simulink model "punto_cd_simulink_200901"  (R2019a)
settings: Solver=VariableStepAuto  StartTime=0.0  StopTime=36*2*pi  RelTol=1e-3
libraries: cstblocks x2
settings Model: Creator=Marco Greco  LastModifiedBy=Marco Greco

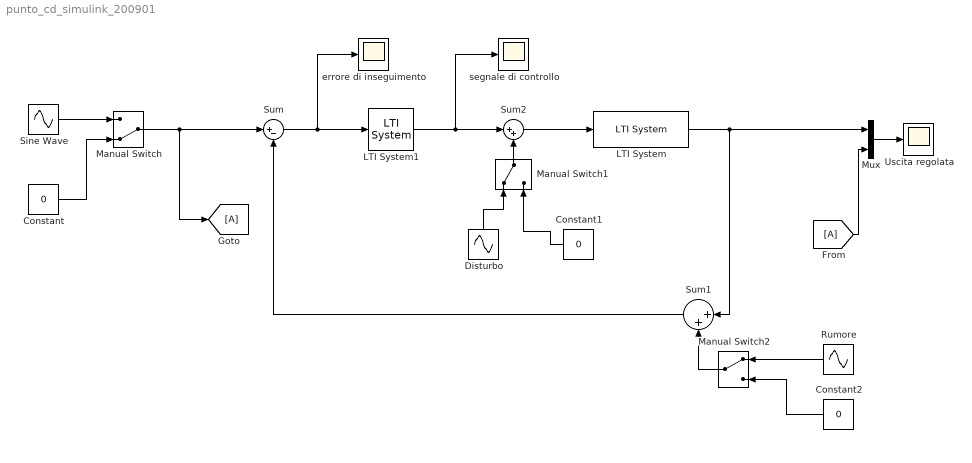
== system punto_cd_simulink_200901 ==
  " Disturbo" : Sin  Frequency=0.2  SampleTime=0
  Constant : Constant  Value=0
  Constant1 : Constant  Value=0
  Constant2 : Constant  Value=0
  LTI System : cstblocks/LTI System  sys=G  IC=[]
  LTI System1 : cstblocks/LTI System  sys=C  IC=[]
  Manual Switch : ManualSwitch  CurrentSetting=0
  Manual Switch1 : ManualSwitch
  Manual Switch2 : ManualSwitch
  Mux : Mux  Inputs=2
  Rumore : Sin  Frequency=60  SampleTime=0
  Sine Wave : Sin  Frequency=1/12  SampleTime=0
  Sum : Sum  Inputs=|+-
  Sum1 : Sum  Inputs=|++
  Sum2 : Sum  Inputs=|++
  Uscita regolata : Scope
  "errore di inseguimento " : Scope
  segnale di controllo : Scope
  wires:
  LTI System1/1 -> Sum2/1, segnale di controllo/1
  Sum/1 -> LTI System1/1, "errore di inseguimento "/1
  [A] -> Mux/2
  Mux/1 -> Uscita regolata/1
  LTI System/1 -> Sum1/1, Mux/1
  Sum1/1 -> Sum/2
  Sum2/1 -> LTI System/1
  Sine Wave/1 -> Manual Switch/1
  Manual Switch/1 -> [A], Sum/1
  Constant/1 -> Manual Switch/2
  Manual Switch1/1 -> Sum2/2
  " Disturbo"/1 -> Manual Switch1/1
  Constant1/1 -> Manual Switch1/2
  Manual Switch2/1 -> Sum1/2
  Rumore/1 -> Manual Switch2/1
  Constant2/1 -> Manual Switch2/2
